simulink model "MODEM_WITH_LOGIC"  (R2021b)
settings: Solver=VariableStepAuto  StartTime=0.0  StopTime=0.002  RelTol=1e-3
libraries: simulink x4, dspsigops x4, dsparch4 x2, commfilt2 x2, dspsrcs4 x1
settings Model: Creator=caccolillo  LastModifiedBy=caccolillo

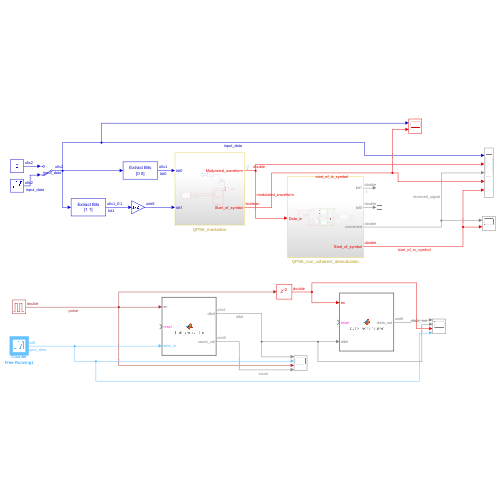
[thumbnail: Simulink's stored preview of the top-level diagram]
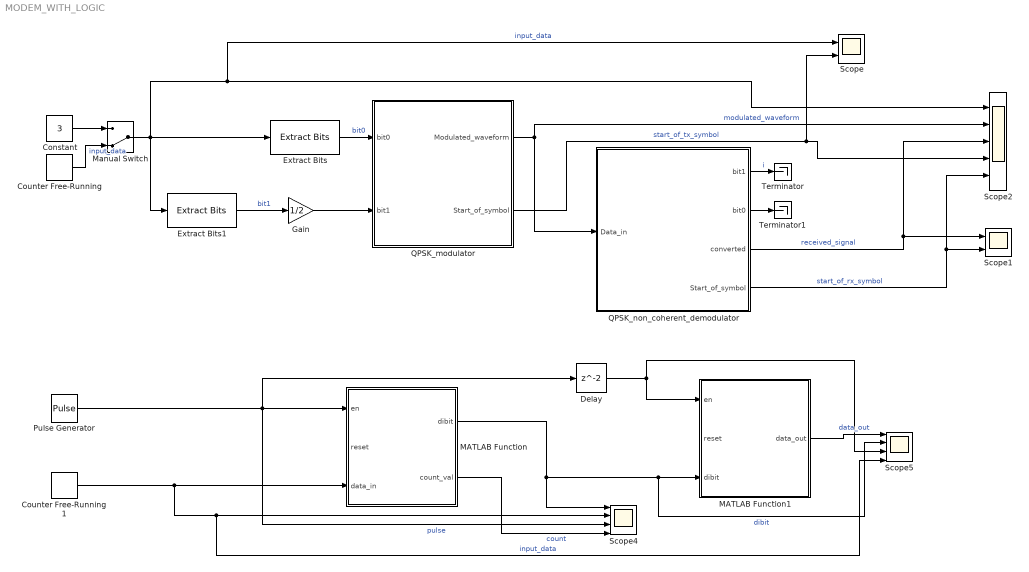
== system MODEM_WITH_LOGIC ==
  Constant : Constant  Value=3  OutDataTypeStr=fixdt(0,2)  SampleTime=1/20000
  Counter Free-Running : simulink/Sources/Counter Free-Running  NumBits=2  tsamp=1/20000
  Counter Free-Running1 : simulink/Sources/Counter Free-Running  NumBits=8  tsamp=4/(20000)
  Delay : Delay
  Extract Bits : simulink/Logic and Bit Operations/Extract Bits  bitsToExtract=Range of bits  numBits=8  bitIdxRange=[0 0]  outScalingMode=Preserve fixed-point scaling
  Extract Bits1 : simulink/Logic and Bit Operations/Extract Bits  bitsToExtract=Range of bits  numBits=8  bitIdxRange=[1 1]  outScalingMode=Preserve fixed-point scaling
  Gain : Gain  Gain=1/2
  MATLAB Function : MATLAB Function  TreatAsAtomicUnit=on
  MATLAB Function1 : MATLAB Function  TreatAsAtomicUnit=on
  Manual Switch : ManualSwitch  CurrentSetting=0
  Pulse Generator : DiscretePulseGenerator  PulseType=Time based  Period=1/20000  PulseWidth=5
  QPSK_modulator : Subsystem
  QPSK_non_coherent_demodulator : Subsystem
  Scope : Scope  NumInputPorts=2
  Scope1 : Scope  NumInputPorts=2
  Scope2 : Scope  NumInputPorts=5
  Scope4 : Scope  NumInputPorts=4
  Scope5 : Scope  NumInputPorts=4
  Terminator : Terminator
  Terminator1 : Terminator
  wires:
  QPSK_modulator/1(Modulated_waveform) -> QPSK_non_coherent_demodulator/1(Data_in), Scope2/2  "modulated_waveform"
  Manual Switch/1 -> Scope/1, Scope2/1, Extract Bits1/1, Extract Bits/1  "input_data"
  Gain/1 -> QPSK_modulator/2(bit1)
  Constant/1 -> Manual Switch/1
  Extract Bits1/1 -> Gain/1  "bit1"
  QPSK_non_coherent_demodulator/3(converted) -> Scope1/1, Scope2/3  "received_signal"
  Counter Free-Running/1 -> Manual Switch/2  "input_data"
  Extract Bits/1 -> QPSK_modulator/1(bit0)  "bit0"
  QPSK_non_coherent_demodulator/1(bit1) -> Terminator/1  "i"
  QPSK_non_coherent_demodulator/2(bit0) -> Terminator1/1
  QPSK_modulator/2(Start_of_symbol) -> Scope/2, Scope2/4  "start_of_tx_symbol"
  QPSK_non_coherent_demodulator/4(Start_of_symbol) -> Scope1/2, Scope2/5  "start_of_rx_symbol"
  MATLAB Function1/1(data_out) -> Scope5/1  "data_out"
  Delay/1 -> MATLAB Function1/1(en), Scope5/3
  Pulse Generator/1 -> Delay/1, Scope4/3, MATLAB Function/1(en)  "pulse"
  MATLAB Function/1(dibit) -> Scope5/2, MATLAB Function1/3(dibit), Scope4/1  "dibit"
  Counter Free-Running1/1 -> Scope5/4, Scope4/2, MATLAB Function/3(data_in)  "input_data"
  MATLAB Function/2(count_val) -> Scope4/4  "count"

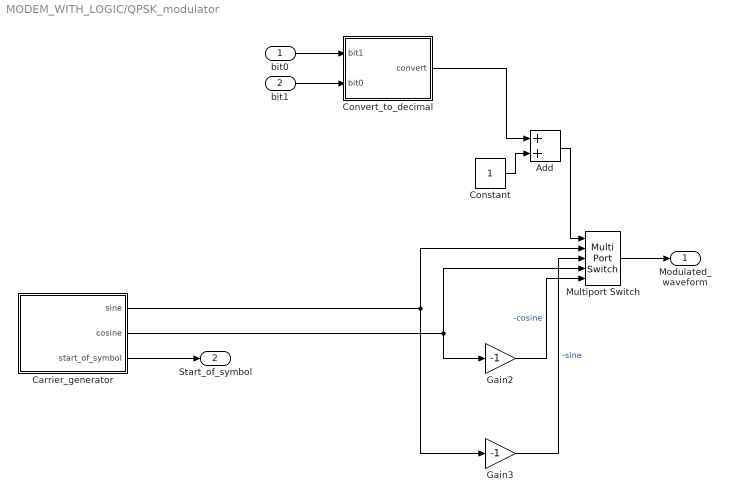
== system MODEM_WITH_LOGIC/QPSK_modulator ==
  bit0 : Inport
  bit1 : Inport  Port=2
  Add : Sum
  Carrier_generator : Subsystem
  Constant : Constant
  Convert_to_decimal : Subsystem
  Gain2 : Gain  Gain=-1
  Gain3 : Gain  Gain=-1
  Multiport Switch : MultiPortSwitch  Inputs=4
  Modulated_waveform : Outport
  Start_of_symbol : Outport  Port=2
  wires:
  Gain3/1 -> Multiport Switch/3  "-sine"
  Multiport Switch/1 -> Modulated_waveform/1
  Gain2/1 -> Multiport Switch/5  "-cosine"
  bit0/1 -> Convert_to_decimal/1(bit1)
  Convert_to_decimal/1(convert) -> Add/1
  Constant/1 -> Add/2
  Add/1 -> Multiport Switch/1
  bit1/1 -> Convert_to_decimal/2(bit0)
  Carrier_generator/2(cosine) -> Gain2/1, Multiport Switch/4
  Carrier_generator/1(sine) -> Gain3/1, Multiport Switch/2
  Carrier_generator/3(start_of_symbol) -> Start_of_symbol/1

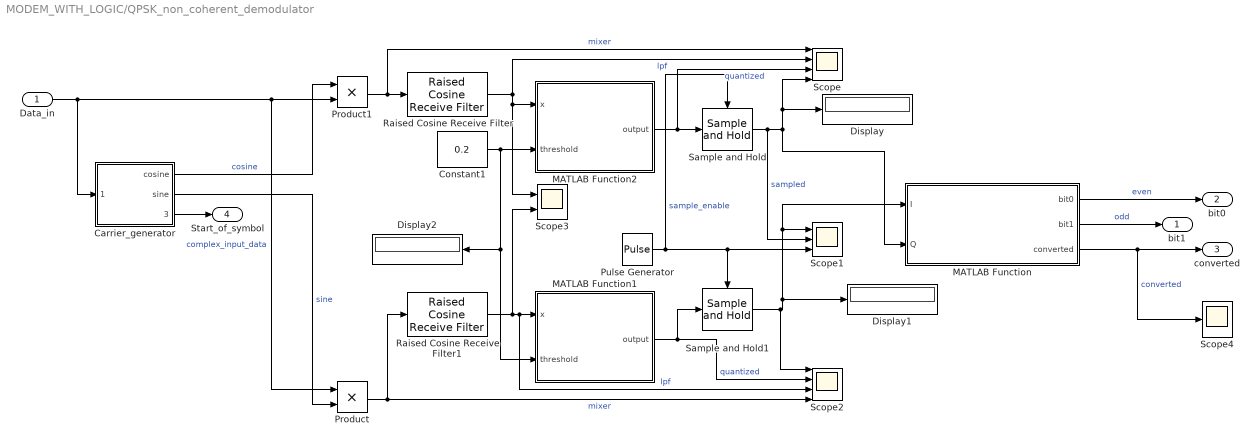
== system MODEM_WITH_LOGIC/QPSK_non_coherent_demodulator ==
  Data_in : Inport
  Carrier_generator : Subsystem
  Constant1 : Constant  Value=0.2
  Display : Display
  Display1 : Display
  Display2 : Display
  MATLAB Function : MATLAB Function  TreatAsAtomicUnit=on
  MATLAB Function1 : MATLAB Function  TreatAsAtomicUnit=on
  MATLAB Function2 : MATLAB Function  TreatAsAtomicUnit=on
  Product : Product
  Product1 : Product
  Pulse Generator : DiscretePulseGenerator  PulseType=Time based  Period=1/20000  PulseWidth=5
  Raised Cosine Receive Filter : commfilt2/Raised Cosine Receive Filter  filtType=Square root  R=0.2  filtSpan=10  N=10  downFactor=2  downOffset=0  filterGain=1  RateOptions=Allow multirate processing  framing=Mute  checkCoeff=off  variableName=rcRxFilt  currentFiltSpan=10  D=5  inputOffset=0  sampMode=Mute  saveAsFlag=0  rateMode=Downsampling  checkGain=Normalized  launchFVT=on  roundingMode=Floor  overflowMode=off  coeffDataTypeStr=Inherit: Same word length as input  coeffMin=[]  coeffMax=[]  coeffLastDataTypeStr=Inherit: Same word length as input  accumDataTypeStr=Inherit: Same as product output  accumLastDataTypeStr=Inherit: Same as product output  outputDataTypeStr=Inherit: Same as accumulator  outputMin=[]  outputMax=[]  outputLastDataTypeStr=Inherit: Same as accumulator
  Raised Cosine Receive Filter1 : commfilt2/Raised Cosine Receive Filter  filtType=Square root  R=0.2  filtSpan=10  N=10  downFactor=2  downOffset=0  filterGain=1  RateOptions=Allow multirate processing  framing=Mute  checkCoeff=off  variableName=rcRxFilt1  currentFiltSpan=10  D=5  inputOffset=0  sampMode=Mute  saveAsFlag=0  rateMode=Downsampling  checkGain=Normalized  launchFVT=on  roundingMode=Floor  overflowMode=off  coeffDataTypeStr=Inherit: Same word length as input  coeffMin=[]  coeffMax=[]  coeffLastDataTypeStr=Inherit: Same word length as input  accumDataTypeStr=Inherit: Same as product output  accumLastDataTypeStr=Inherit: Same as product output  outputDataTypeStr=Inherit: Same as accumulator  outputMin=[]  outputMax=[]  outputLastDataTypeStr=Inherit: Same as accumulator
  Sample and Hold : dspsigops/Sample and Hold  trig=Rising edge  initCond=0  latchinput=off
  Sample and Hold1 : dspsigops/Sample and Hold  trig=Rising edge  initCond=0  latchinput=off
  Scope : Scope  NumInputPorts=4
  Scope1 : Scope  NumInputPorts=3
  Scope2 : Scope  NumInputPorts=4
  Scope3 : Scope  NumInputPorts=2
  Scope4 : Scope
  bit1 : Outport
  bit0 : Outport  Port=2
  converted : Outport  Port=3
  Start_of_symbol : Outport  Port=4
  wires:
  Data_in/1 -> Product/1, Product1/2, Carrier_generator/1(Modulated_signal)  "complex_input_data"
  Product1/1 -> Raised Cosine Receive Filter/1, Scope/1  "mixer"
  Raised Cosine Receive Filter/1 -> MATLAB Function2/1(x), Scope3/1, Scope/2  "lpf"
  Product/1 -> Raised Cosine Receive Filter1/1, Scope2/4  "mixer"
  Pulse Generator/1 -> Sample and Hold1/Trigger, Scope1/3, Sample and Hold/Trigger  "sample_enable"
  MATLAB Function1/1(output) -> Scope2/2, Sample and Hold1/1  "quantized"
  Sample and Hold/1 -> MATLAB Function/2(Q), Scope/4, Display/1, Scope1/2  "sampled"
  MATLAB Function2/1(output) -> Scope/3, Sample and Hold/1  "quantized"
  Carrier_generator/2(sine) -> Product/2  "sine"
  Sample and Hold1/1 -> Display1/1, MATLAB Function/1(I), Scope1/1, Scope2/1
  Carrier_generator/1(cosine) -> Product1/1  "cosine"
  Raised Cosine Receive Filter1/1 -> Scope2/3, MATLAB Function1/1(x), Scope3/2  "lpf"
  MATLAB Function/1(bit0) -> bit0/1  "even"
  MATLAB Function/2(bit1) -> bit1/1  "odd"
  MATLAB Function/3(converted) -> converted/1, Scope4/1  "converted"
  Constant1/1 -> Display2/1, MATLAB Function1/2(threshold), MATLAB Function2/2(threshold)
  Carrier_generator/3(start_of_symbol) -> Start_of_symbol/1

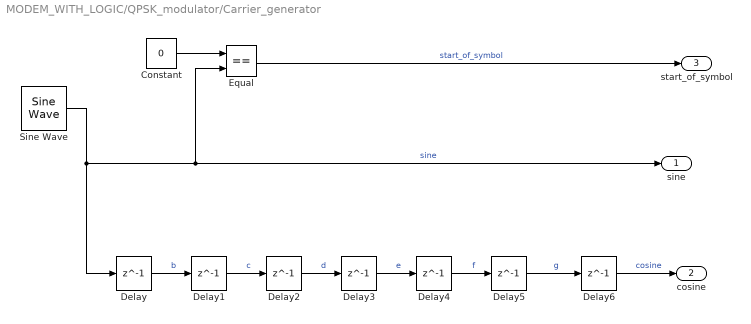
== system MODEM_WITH_LOGIC/QPSK_modulator/Carrier_generator ==
  Constant : Constant  Value=0
  Delay{,1..6} (7 alike) : Delay  DelayLength=1  InitialCondition=0
  Equal : RelationalOperator  Operator===  OutDataTypeStr=boolean  RndMeth=Simplest
  Sine Wave : dspsrcs4/Sine Wave  Amplitude=1  Frequency=20000  Phase=0  SampleMode=Discrete  OutComplex=Real  CompMethod=Table lookup  TableSize=Speed  SampleTime=1/200000  SamplesPerFrame=1  ResetState=Restart at time zero  OutputFrames=off  dataType=double  wordLen=16  udDataType=sfix(16)  fracBitsMode=Best precision  numFracBits=15  OutDataTypeStr=double  LastOutDataTypeStr=double
  sine : Outport
  cosine : Outport  Port=2
  start_of_symbol : Outport  Port=3
  wires:
  Delay/1 -> Delay1/1  "b"
  Delay2/1 -> Delay3/1  "d"
  Delay6/1 -> cosine/1  "cosine"
  Sine Wave/1 -> Equal/2, sine/1, Delay/1  "sine"
  Delay5/1 -> Delay6/1  "g"
  Delay3/1 -> Delay4/1  "e"
  Delay4/1 -> Delay5/1  "f"
  Delay1/1 -> Delay2/1  "c"
  Constant/1 -> Equal/1
  Equal/1 -> start_of_symbol/1  "start_of_symbol"

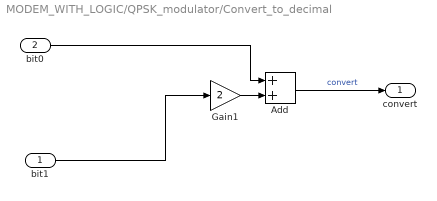
== system MODEM_WITH_LOGIC/QPSK_modulator/Convert_to_decimal ==
  bit1 : Inport
  bit0 : Inport  Port=2
  Add : Sum
  Gain1 : Gain  Gain=2
  convert : Outport
  wires:
  bit1/1 -> Gain1/1
  bit0/1 -> Add/1
  Add/1 -> convert/1  "convert"
  Gain1/1 -> Add/2

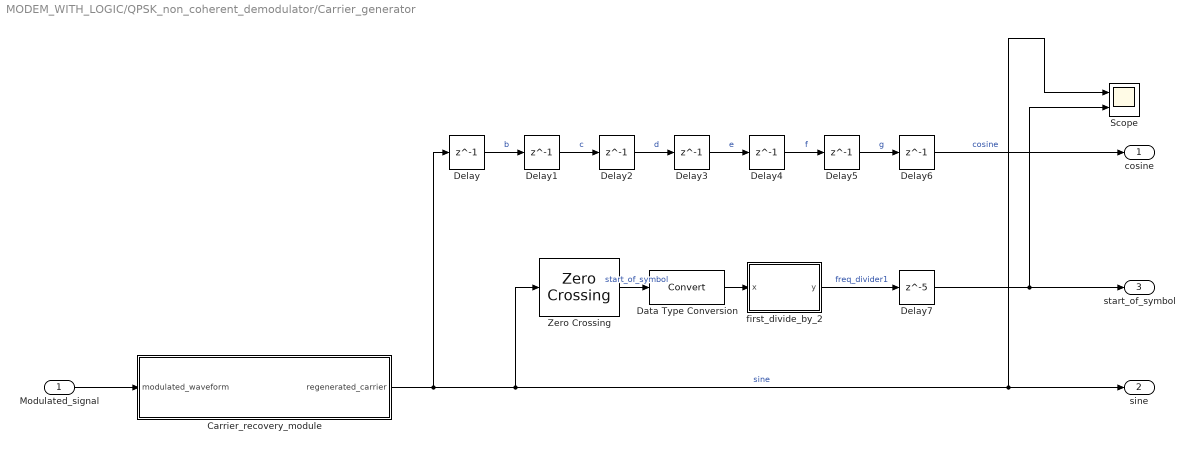
== system MODEM_WITH_LOGIC/QPSK_non_coherent_demodulator/Carrier_generator ==
  Modulated_signal : Inport
  Carrier_recovery_module : Subsystem
  Data Type Conversion : DataTypeConversion
  Delay{,1..6} (7 alike) : Delay  DelayLength=1  InitialCondition=0
  Delay7 : Delay  DelayLength=5
  Scope : Scope  NumInputPorts=2
  Zero Crossing : dspsigops/Zero Crossing  InputProcessing=Columns as channels (frame based)
      settings: SourceProductBaseCode=DS
  first_divide_by_2 : MATLAB Function  TreatAsAtomicUnit=on
  cosine : Outport
  sine : Outport  Port=2
  start_of_symbol : Outport  Port=3
  wires:
  Delay1/1 -> Delay2/1  "c"
  Delay5/1 -> Delay6/1  "g"
  Delay2/1 -> Delay3/1  "d"
  Delay6/1 -> cosine/1  "cosine"
  Delay3/1 -> Delay4/1  "e"
  Delay/1 -> Delay1/1  "b"
  Delay4/1 -> Delay5/1  "f"
  Modulated_signal/1 -> Carrier_recovery_module/1(modulated_waveform)
  Zero Crossing/1 -> Data Type Conversion/1  "start_of_symbol"
  Carrier_recovery_module/1(regenerated_carrier) -> Delay/1, Scope/1, sine/1, Zero Crossing/1  "sine"
  first_divide_by_2/1(y) -> Delay7/1  "freq_divider1"
  Data Type Conversion/1 -> first_divide_by_2/1(x)
  Delay7/1 -> Scope/2, start_of_symbol/1

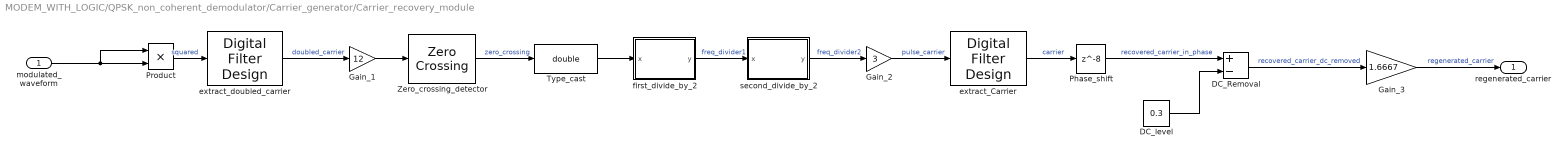
== system MODEM_WITH_LOGIC/QPSK_non_coherent_demodulator/Carrier_generator/Carrier_recovery_module ==
  modulated_waveform : Inport
  DC_Removal : Sum  Inputs=+-
  DC_level : Constant  Value=0.3
  Gain_1 : Gain  Gain=12
  Gain_2 : Gain  Gain=3
  Gain_3 : Gain  Gain=1.6667
  Phase_shift : Delay  DelayLength=8
  Product : Product
  Type_cast : DataTypeConversion  OutDataTypeStr=double
  Zero_crossing_detector : dspsigops/Zero Crossing  InputProcessing=Columns as channels (frame based)
      settings: SourceProductBaseCode=DS
  extract_Carrier : dsparch4/Digital Filter Design  mwdsp_browser_bugfix_var=off
  extract_doubled_carrier : dsparch4/Digital Filter Design  mwdsp_browser_bugfix_var=off
  first_divide_by_2 : MATLAB Function  TreatAsAtomicUnit=on
  second_divide_by_2 : MATLAB Function  TreatAsAtomicUnit=on
  regenerated_carrier : Outport
  wires:
  modulated_waveform/1 -> Product/1, Product/2
  DC_level/1 -> DC_Removal/2
  Gain_3/1 -> regenerated_carrier/1  "regenerated_carrier"
  Phase_shift/1 -> DC_Removal/1  "recovered_carrier_in_phase"
  DC_Removal/1 -> Gain_3/1  "recovered_carrier_dc_removed"
  Product/1 -> extract_doubled_carrier/1  "squared"
  extract_doubled_carrier/1 -> Gain_1/1  "doubled_carrier"
  Gain_2/1 -> extract_Carrier/1  "pulse_carrier"
  second_divide_by_2/1(y) -> Gain_2/1  "freq_divider2"
  first_divide_by_2/1(y) -> second_divide_by_2/1(x)  "freq_divider1"
  Gain_1/1 -> Zero_crossing_detector/1
  Type_cast/1 -> first_divide_by_2/1(x)
  extract_Carrier/1 -> Phase_shift/1  "carrier"
  Zero_crossing_detector/1 -> Type_cast/1  "zero_crossing"

== matlab function MODEM_WITH_LOGIC/QPSK_non_coherent_demodulator/MATLAB Function1 ==
  data: x input; output output; threshold input
function output = discretize_input(x,threshold)
    if x > threshold
        output = 1;
    else
        output = 0;
    end
end

== matlab function MODEM_WITH_LOGIC/QPSK_non_coherent_demodulator/MATLAB Function2 ==
  data: x input; output output; threshold input
function output = discretize_input(x,threshold)
    if x > threshold
        output = 1;
    else
        output = 0;
    end
end

== matlab function MODEM_WITH_LOGIC/QPSK_non_coherent_demodulator/Carrier_generator/Carrier_recovery_module/first_divide_by_2 ==
  data: x input; y output
function y = freqDivider(x)
% freqDivider  Frequency divider using persistent 2-sample input buffer
%
%   y = freqDivider(x) processes a single input sample x (scalar), and
%   returns a scalar output y, which goes high on every second rising edge.
%
%   This function is stateful and maintains internal buffer and edge counter
%   across calls using persistent variables.

    % Declare persistent variables
    persistent buf riseCount

    % Initialize persistent variables on first call
    if isempty(buf)
        buf = [0, 0];      % input buffer: [x(i-2), x(i-1)]
        riseCount = 0;     % rising edge counter
    end

    % Shift input buffer
    buf = [buf(2), x];

    % Default output
    y = 0;

    % Detect rising edge: x(i-1) <= 0 and x(i) > 0
    if buf(1) <= 0 && buf(2) > 0
        riseCount = riseCount + 1;

        if mod(riseCount, 2) == 0
            y = 1;  % Output high on every 2nd rising edge
        end
    end
end

== matlab function MODEM_WITH_LOGIC/QPSK_non_coherent_demodulator/MATLAB Function ==
  data: bit0 output; I input; bit1 output; Q input; converted output
function [bit0, bit1,converted] = qpsk_demod_scalar(I, Q)
%QPSK_DEMOD_SCALAR Demodulates one QPSK symbol (scalar I/Q) into two bits.
% Inputs:
%   I - In-phase component (scalar)
%   Q - Quadrature component (scalar)
% Outputs:
%   bit1 - First bit (MSB)
%   bit2 - Second bit (LSB)

    % QPSK Gray demapping
    if I == 1 && Q == 1
        bit0 = 0; bit1 = 0;
        converted = 0;
    elseif I == 0 && Q == 1
        bit0 = 0; bit1 = 1;
        converted = 1;
    elseif I == 0 && Q == 0
        bit0 = 0; bit1 = 1;
        converted = 2;
    elseif I == 1 && Q == 0
        bit0 = 1; bit1 = 1;
        converted = 3;
    else
        % Edge case: I or Q == 0 (treat as 0)
        bit0 = 0;
        bit1 = 0;
        converted = 0;
    end
end

== matlab function MODEM_WITH_LOGIC/QPSK_non_coherent_demodulator/Carrier_generator/Carrier_recovery_module/second_divide_by_2 ==
  data: x input; y output
function y = freqDivider(x)
% freqDivider  Frequency divider using persistent 2-sample input buffer
%
%   y = freqDivider(x) processes a single input sample x (scalar), and
%   returns a scalar output y, which goes high on every second rising edge.
%
%   This function is stateful and maintains internal buffer and edge counter
%   across calls using persistent variables.

    % Declare persistent variables
    persistent buf riseCount

    % Initialize persistent variables on first call
    if isempty(buf)
        buf = [0, 0];      % input buffer: [x(i-2), x(i-1)]
        riseCount = 0;     % rising edge counter
    end

    % Shift input buffer
    buf = [buf(2), x];

    % Default output
    y = 0;

    % Detect rising edge: x(i-1) <= 0 and x(i) > 0
    if buf(1) <= 0 && buf(2) > 0
        riseCount = riseCount + 1;

        if mod(riseCount, 2) == 0
            y = 1;  % Output high on every 2nd rising edge
        end
    end
end

== matlab function MODEM_WITH_LOGIC/QPSK_non_coherent_demodulator/Carrier_generator/first_divide_by_2 ==
  data: x input; y output
function y = freqDivider(x)
% freqDivider  Frequency divider using persistent 2-sample input buffer
%
%   y = freqDivider(x) processes a single input sample x (scalar), and
%   returns a scalar output y, which goes high on every second rising edge.
%
%   This function is stateful and maintains internal buffer and edge counter
%   across calls using persistent variables.

    % Declare persistent variables
    persistent buf riseCount

    % Initialize persistent variables on first call
    if isempty(buf)
        buf = [0, 0];      % input buffer: [x(i-2), x(i-1)]
        riseCount = 0;     % rising edge counter
    end

    % Shift input buffer
    buf = [buf(2), x];

    % Default output
    y = 0;

    % Detect rising edge: x(i-1) <= 0 and x(i) > 0
    if buf(1) <= 0 && buf(2) > 0
        riseCount = riseCount + 1;

        if mod(riseCount, 2) == 0
            y = 1;  % Output high on every 2nd rising edge
        end
    end
end

== matlab function MODEM_WITH_LOGIC/MATLAB Function ==
  data: en input; dibit output; reset input; data_in input; count_val output
function [dibit,count_val] = dibit_extractor(en, reset, data_in)
% dibit_extractor  Extracts two-bit segments from an 8-bit input on enable pulses
%   en      : boolean enable signal (rising edge triggers output update)
%   reset   : boolean reset signal (synchronous reset of internal state)
%   data_in : uint8 8-bit input data
%   dibit   : UFix_2_0 2-bit unsigned fixed-point output

%#codegen

persistent count prev_en
if isempty(count)
    count   = uint8(3);   % cycle index (0 to 3)
    prev_en = 0;       % previous enable state
end

% Synchronous reset
if reset
    count = uint8(0);
end

% Detect rising edge of enable
if en==1 && prev_en==0 && ~reset
    % Increment and wrap count
    count = mod(count + 1, 4);
end
prev_en = en;

% Determine starting bit position (0-based)
startBit = count * 2;

% Extract two bits (MATLAB bitget uses 1-based positions)
bit0 = bitget(data_in, startBit + 1);
bit1 = bitget(data_in, startBit + 2);

% Assemble value (bit1 is MSB, bit0 is LSB)
value = uint8(bit1) * 2 + uint8(bit0);

% Create 2-bit unsigned fixed-point output
dibit = fi(value, 0, 2, 0);
count_val = count
end

== matlab function MODEM_WITH_LOGIC/MATLAB Function1 ==
  data: en input; data_out output; reset input; dibit input
function data_out = byte_assembler(en, reset, dibit)
% byte_assembler  Assembles 8-bit data from four 2-bit segments
%   en        : boolean enable signal (rising edge triggers input sampling)
%   reset     : boolean reset signal (synchronous reset of internal state)
%   dibit     : ufix2 2-bit input
%   data_out  : uint8 8-bit output, valid after 4 dibits

%#codegen

persistent count temp_byte prev_en
if isempty(count)
    count = uint8(0);
    temp_byte = uint8(0);
    prev_en = 0;
end

% Synchronous reset
if reset
    count = uint8(0);
    temp_byte = uint8(0);
end

% Detect rising edge of enable
if en==1 && prev_en==0 && ~reset
    shift = bitshift(uint8(dibit), count * 2);  % Place dibit at the correct position
    mask = bitshift(uint8(3), count * 2);       % Create mask for clearing that position
    temp_byte = bitor(bitand(temp_byte, bitcmp(mask, 'uint8')), shift);

    % Increment count and wrap
    count = mod(count + 1, 4);
end
prev_en = en;

% Output the assembled byte only when 4 dibits have been collected
if count == 0 && ~reset
    data_out = temp_byte;
else
    data_out = uint8(0);
end
end
